simulink model "adsl_sim"  (Simulink 6.0)
settings: Solver=ode45  SolverMode=SingleTasking  StartTime=0.0  StopTime=2  RelTol=1e-3
PreLoadFcn:
  | % variables are initialized through the Model Workspace
model workspace: external: M-Code (data not in the file)
values from neighbouring files (symbols this model uses):
  H = conv2(chCoeff',W)    [eq_computecostfcn.m]
undefined symbols (not defined in the file or in its folder): b, rsgenpoly, slcm
libraries: commdigbbndam2 x512, simulink x37, commutil2 x8, commblkcod2 x4, commsequence2 x4, commsink2 x4, commcrc2 x4, commcnvintrlv2 x2, dspxfrm3 x2, dspsrcs4 x2, dspsigattribs x1, dspmtrx3 x1
(part 1 of 5)
Description:
  | 256 Channel Discrete Multi-Tone Signaling as used in ADSL
CloseFcn:
  | clear adslSigsOut
  | clear global GF_TABLE1 GF_TABLE2 GF_TABLE_M GF_TABLE_PRIM_POLY
settings Model: CovMetricSettings=d  Creator=mikem  LastModifiedBy=akansal  ExtModeAutoUpdateStatusClock=off  BufferReuse=off  ProdHWDeviceType=Specified
settings DataIOCC: SaveOutput=off  SaveTime=off  SignalLoggingName=adslSigsOut
settings OptimizationCC: BlockReduction=off  BooleanDataType=off  OptimizeBlockIOStorage=off  BufferReuse=off  LocalBlockOutputs=off
settings DebuggingCC: CheckExecutionContextPreStartOutputMsg=on  CheckExecutionContextRuntimeOutputMsg=on  SolverPrmCheckMsg=none
settings HardwareCC: ProdHWDeviceType=Specified
settings ModelReferenceCC: UpdateModelReferenceTargets=IfOutOfDate
settings GRTTargetCC: LifeSpan=inf
settings SFSimCC: SFSimApplyToAllLibs=on  SFSimBuildMode=Incremental

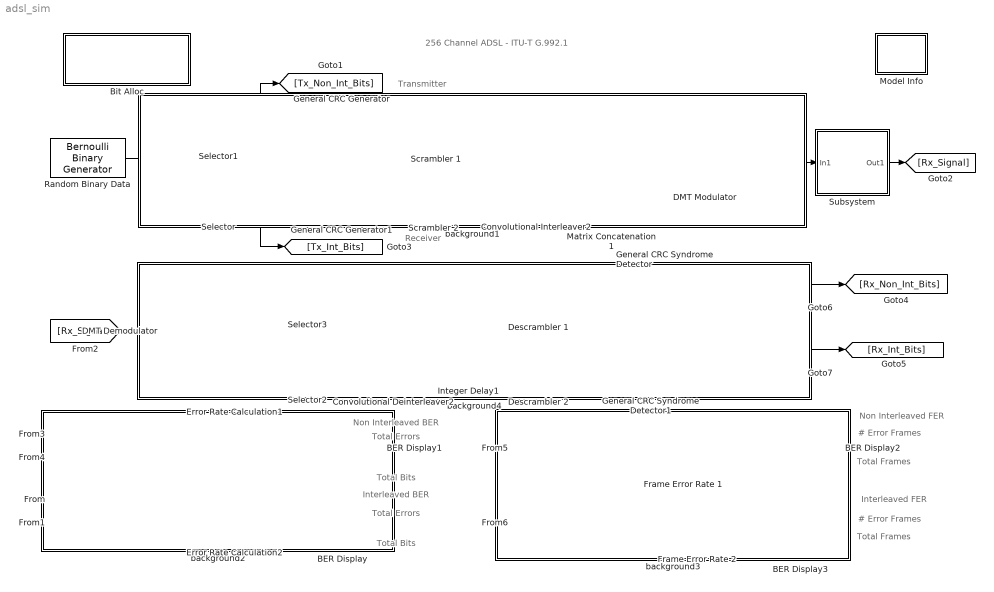
== system adsl_sim ==
  note: Transmitter
  note: Receiver
  note: 256 Channel ADSL - ITU-T G.992.1
  note: Total Bits
  note: Total Errors
  note: Non Interleaved BER
  note: Total Bits
  note: Total Errors
  note: Interleaved BER
  note: # Error Frames
  note: Total Frames
  note: Interleaved FER
  note: # Error Frames
  note: Total Frames
  note: Non Interleaved FER
  BER Display{,1..3} (4 alike) : Display
  Bit Alloc : Subsystem  EnableExecutionContextPropagation=on
      settings: OpenFcn=load('bit_allocation'),plot(b),axis([0 257 1 11]),title('Bit Allocations'),xlabel('Channel'),ylabel('No. Bits')
      mask Display: disp('Load and Plot\nBit Allocation Vector')
  Convolutional Deinterleaver2 : commcnvintrlv2/Convolutional Deinterleaver  N=5  B=2  ic=0
  Convolutional Interleaver2 : commcnvintrlv2/Convolutional Interleaver  N=5  B=2  ic=0
  DMT Demodulator : Subsystem  EnableExecutionContextPropagation=on
      mask Display: disp('DMT\nDemodulator')
  DMT Modulator : Subsystem  EnableExecutionContextPropagation=on
      mask Display: disp('DMT\nModulator')
  Descrambler 1 : Subsystem  EnableExecutionContextPropagation=on
      mask Display: disp('Descrambler\n & FEC');
  Descrambler 2 : Subsystem  EnableExecutionContextPropagation=on
      mask Display: disp('Descrambler\n & FEC');
  Error Rate Calculation1 : commsink2/Error Rate Calculation  N=0  st_delay=0  cp_mode=Entire frame  subframe=[]  PMode=Port  WsName=ErrorVec  RsMode2=off  stop=off  numErr=100  maxBits=1000
  Error Rate Calculation2 : commsink2/Error Rate Calculation  N=776  st_delay=0  cp_mode=Entire frame  subframe=[]  PMode=Port  WsName=ErrorVec  RsMode2=off  stop=off  numErr=100  maxBits=1000
  Frame Error Rate 1 : Subsystem  EnableExecutionContextPropagation=on
      mask Display: disp('Frame Error Rate\n Calculation');
  Frame Error Rate 2 : Subsystem  EnableExecutionContextPropagation=on
      mask Display: disp('Frame Error Rate\n Calculation');
  General CRC Generator : commcrc2/General CRC Generator  genPoly=[1 0 0 0 1 1 1 0 1]  iniStates=[0]  numChecksums=1
  General CRC Generator1 : commcrc2/General CRC Generator  genPoly=[1 0 0 0 1 1 1 0 1]  iniStates=[0]  numChecksums=1
  General CRC Syndrome Detector : commcrc2/General CRC Syndrome Detector  genPoly=[1 0 0 0 1 1 1 0 1]  iniStates=[0]  numChecksums=1
  General CRC Syndrome Detector1 : commcrc2/General CRC Syndrome Detector  genPoly=[1 0 0 0 1 1 1 0 1]  iniStates=[0]  numChecksums=1
  Integer Delay1 : dspsigops/Delay  dly_unit=Samples  delay=800  ic_detail=off  dif_ic_for_ch=off  dif_ic_for_dly=off  ic=0  reset_popup=None
  Matrix Concatenation1 : simulink/Math Operations/Matrix Concatenation  numInports=2  catMethod=Vertical
  Model Info : Subsystem  LoadFcn=slcm LoadBlock;  InitFcn=slcm('UpdateAllCMBlocksInThisModelInit')  EnableExecutionContextPropagation=on  mask(CMBlock){InitialSaveTempField=, InitialBlockCM=none, BlockCM=none, Frame=on, SaveTempField=, DisplayStringWithTags=Info, MaskDisplayString=Info, HorizontalTextAlignment=Center, LeftAlignmentValue=0.5, SourceBlockDiagram=adsl_sim, TagMaxNumber=20, CMTag1=, CMTag2=, CMTag3=, CMTag4=, CMTag5=, CMTag6=, CMTag7=, CMTag8=, CMTag9=, CMTag10=, CMTag11=, CMTag12=, CMTag13=, CMTag14=, CMTag15=, CMTag16=, CMTag17=, CMTag18=, CMTag19=, CMTag20=}
      mask help: This block allows revision control information to be displayed within the model.
      settings: CopyFcn=slcm CopyBlock;  DeleteFcn=slcm Cancel;  PostSaveFcn=slcm('UpdateAllCMBlocksInThisModel')  NameChangeFcn=slcm Rename;  OpenFcn=commdemohelp;
      mask Display: text(str2num(LeftAlignmentValue), 0.5, MaskDisplayString, 'HorizontalAlignment', HorizontalTextAlignment)
  Random Binary Data : commrandsrc2/Bernoulli Binary Generator  P=0.5  seed=4321  Ts=(1/4000)/1552  frameBased=on  sampPerFrame=1552  orient=off
  Scrambler 1 : Subsystem  EnableExecutionContextPropagation=on
      mask Display: disp('Scrambler\n & FEC');
  Scrambler 2 : Subsystem  EnableExecutionContextPropagation=on
      mask Display: disp('Scrambler \n & FEC');
  Selector : Selector  Elements=[777:1552]  InputPortWidth=1552
  Selector1 : Selector  Elements=[1:776]  InputPortWidth=1552
  Selector2 : Selector  Elements=[841:1680]  InputPortWidth=1680
  Selector3 : Selector  Elements=[1:840]  InputPortWidth=1680
  Subsystem : Subsystem  EnableExecutionContextPropagation=on
      mask Type: telchannel
      mask Display: disp('Telephone\nLine');
  background1 : Subsystem  EnableExecutionContextPropagation=on
      mask Display: disp('')
  background2 : Subsystem  EnableExecutionContextPropagation=on
      mask Display: disp('')
  background3 : Subsystem  EnableExecutionContextPropagation=on
      mask Display: disp('')
  background4 : Subsystem  EnableExecutionContextPropagation=on
      mask Display: disp('')
  wires:
  Error Rate Calculation2/1 -> BER Display/1
  DMT Modulator/1(Out) -> Subsystem/1(In1)
  Scrambler 1/1(Out1) -> Matrix Concatenation1/1
  Matrix Concatenation1/1 -> DMT Modulator/1(In)
  Selector3/1 -> Descrambler 1/1(In1)
  Scrambler 2/1(Out1) -> Convolutional Interleaver2/1
  Convolutional Interleaver2/1 -> Matrix Concatenation1/2
  Selector2/1 -> Convolutional Deinterleaver2/1
  Convolutional Deinterleaver2/1 -> Integer Delay1/1
  General CRC Generator1/1 -> Scrambler 2/1(In1)
  Selector/1 -> [Tx_Int_Bits], General CRC Generator1/1
  Selector1/1 -> [Tx_Non_Int_Bits], General CRC Generator/1
  General CRC Generator/1 -> Scrambler 1/1(In1)
  General CRC Syndrome Detector/1 -> [Rx_Non_Int_Bits]
  General CRC Syndrome Detector1/1 -> [Rx_Int_Bits]
  Descrambler 2/1(Out1) -> General CRC Syndrome Detector1/1
  Descrambler 1/1(Out1) -> General CRC Syndrome Detector/1
  General CRC Syndrome Detector1/2 -> [CRC_syndrome2]
  General CRC Syndrome Detector/2 -> [CRC_syndrome1]
  [Tx_Int_Bits] -> Error Rate Calculation2/1
  [Rx_Int_Bits] -> Error Rate Calculation2/2
  Subsystem/1(Out1) -> [Rx_Signal]
  [Rx_Signal] -> DMT Demodulator/1(In)
  Random Binary Data/1 -> Selector/1, Selector1/1
  Error Rate Calculation1/1 -> BER Display1/1
  [Tx_Non_Int_Bits] -> Error Rate Calculation1/1
  [Rx_Non_Int_Bits] -> Error Rate Calculation1/2
  DMT Demodulator/1(Out) -> Selector3/1, Selector2/1
  Frame Error Rate 1/1(Out1) -> BER Display2/1
  [CRC_syndrome1] -> Frame Error Rate 1/1(In1)
  Frame Error Rate 2/1(Out1) -> BER Display3/1
  [CRC_syndrome2] -> Frame Error Rate 2/1(In1)
  Integer Delay1/1 -> Descrambler 2/1(In1)

== system adsl_sim/Bit Alloc ==

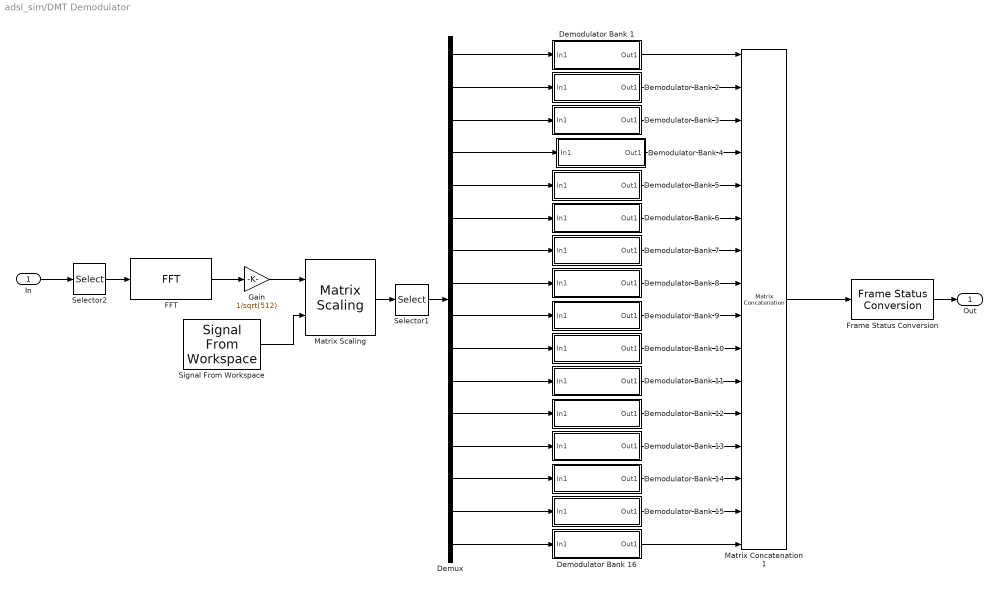
== system adsl_sim/DMT Demodulator ==
  In : Inport  LatchInput=off
  Demodulator Bank 1 : Subsystem  EnableExecutionContextPropagation=on  mask(Demodulator Bank){offset=16*0}
      mask prompts: offset "Index offset:"
      mask help: Bank of sixteen demodulators for use in DMT. Each demodulator in the bank is a Rectangular QAM demodulator. The M-ary number for each demodulator is taken from a workspace variable b. The Index offset parameter determines which sixteen consecutive values from b to use for this bank of demodulators.
      mask Display: disp('Demodulator\nBank');
  Demodulator Bank 10 : Subsystem  EnableExecutionContextPropagation=on  mask(Demodulator Bank){offset=16*9}
      mask prompts: offset "Index offset:"
      mask help: Bank of sixteen demodulators for use in DMT. Each demodulator in the bank is a Rectangular QAM demodulator. The M-ary number for each demodulator is taken from a workspace variable b. The Index offset parameter determines which sixteen consecutive values from b to use for this bank of demodulators.
      mask Display: disp('Demodulator\nBank');
  Demodulator Bank 11 : Subsystem  EnableExecutionContextPropagation=on  mask(Demodulator Bank){offset=16*10}
      mask prompts: offset "Index offset:"
      mask help: Bank of sixteen demodulators for use in DMT. Each demodulator in the bank is a Rectangular QAM demodulator. The M-ary number for each demodulator is taken from a workspace variable b. The Index offset parameter determines which sixteen consecutive values from b to use for this bank of demodulators.
      mask Display: disp('Demodulator\nBank');
  Demodulator Bank 12 : Subsystem  EnableExecutionContextPropagation=on  mask(Demodulator Bank){offset=16*11}
      mask prompts: offset "Index offset:"
      mask help: Bank of sixteen demodulators for use in DMT. Each demodulator in the bank is a Rectangular QAM demodulator. The M-ary number for each demodulator is taken from a workspace variable b. The Index offset parameter determines which sixteen consecutive values from b to use for this bank of demodulators.
      mask Display: disp('Demodulator\nBank');
  Demodulator Bank 13 : Subsystem  EnableExecutionContextPropagation=on  mask(Demodulator Bank){offset=16*12}
      mask prompts: offset "Index offset:"
      mask help: Bank of sixteen demodulators for use in DMT. Each demodulator in the bank is a Rectangular QAM demodulator. The M-ary number for each demodulator is taken from a workspace variable b. The Index offset parameter determines which sixteen consecutive values from b to use for this bank of demodulators.
      mask Display: disp('Demodulator\nBank');
  Demodulator Bank 14 : Subsystem  EnableExecutionContextPropagation=on  mask(Demodulator Bank){offset=16*13}
      mask prompts: offset "Index offset:"
      mask help: Bank of sixteen demodulators for use in DMT. Each demodulator in the bank is a Rectangular QAM demodulator. The M-ary number for each demodulator is taken from a workspace variable b. The Index offset parameter determines which sixteen consecutive values from b to use for this bank of demodulators.
      mask Display: disp('Demodulator\nBank');
  Demodulator Bank 15 : Subsystem  EnableExecutionContextPropagation=on  mask(Demodulator Bank){offset=16*14}
      mask prompts: offset "Index offset:"
      mask help: Bank of sixteen demodulators for use in DMT. Each demodulator in the bank is a Rectangular QAM demodulator. The M-ary number for each demodulator is taken from a workspace variable b. The Index offset parameter determines which sixteen consecutive values from b to use for this bank of demodulators.
      mask Display: disp('Demodulator\nBank');
  Demodulator Bank 16 : Subsystem  EnableExecutionContextPropagation=on  mask(Demodulator Bank){offset=16*15}
      mask prompts: offset "Index offset:"
      mask help: Bank of sixteen demodulators for use in DMT. Each demodulator in the bank is a Rectangular QAM demodulator. The M-ary number for each demodulator is taken from a workspace variable b. The Index offset parameter determines which sixteen consecutive values from b to use for this bank of demodulators.
      mask Display: disp('Demodulator\nBank');
  Demodulator Bank 2 : Subsystem  EnableExecutionContextPropagation=on  mask(Demodulator Bank){offset=16*1}
      mask prompts: offset "Index offset:"
      mask help: Bank of sixteen demodulators for use in DMT. Each demodulator in the bank is a Rectangular QAM demodulator. The M-ary number for each demodulator is taken from a workspace variable b. The Index offset parameter determines which sixteen consecutive values from b to use for this bank of demodulators.
      mask Display: disp('Demodulator\nBank');
  Demodulator Bank 3 : Subsystem  EnableExecutionContextPropagation=on  mask(Demodulator Bank){offset=16*2}
      mask prompts: offset "Index offset:"
      mask help: Bank of sixteen demodulators for use in DMT. Each demodulator in the bank is a Rectangular QAM demodulator. The M-ary number for each demodulator is taken from a workspace variable b. The Index offset parameter determines which sixteen consecutive values from b to use for this bank of demodulators.
      mask Display: disp('Demodulator\nBank');
  Demodulator Bank 4 : Subsystem  EnableExecutionContextPropagation=on  mask(Demodulator Bank){offset=16*3}
      mask prompts: offset "Index offset:"
      mask help: Bank of sixteen demodulators for use in DMT. Each demodulator in the bank is a Rectangular QAM demodulator. The M-ary number for each demodulator is taken from a workspace variable b. The Index offset parameter determines which sixteen consecutive values from b to use for this bank of demodulators.
      mask Display: disp('Demodulator\nBank');
  Demodulator Bank 5 : Subsystem  EnableExecutionContextPropagation=on  mask(Demodulator Bank){offset=16*4}
      mask prompts: offset "Index offset:"
      mask help: Bank of sixteen demodulators for use in DMT. Each demodulator in the bank is a Rectangular QAM demodulator. The M-ary number for each demodulator is taken from a workspace variable b. The Index offset parameter determines which sixteen consecutive values from b to use for this bank of demodulators.
      mask Display: disp('Demodulator\nBank');
  Demodulator Bank 6 : Subsystem  EnableExecutionContextPropagation=on  mask(Demodulator Bank){offset=16*5}
      mask prompts: offset "Index offset:"
      mask help: Bank of sixteen demodulators for use in DMT. Each demodulator in the bank is a Rectangular QAM demodulator. The M-ary number for each demodulator is taken from a workspace variable b. The Index offset parameter determines which sixteen consecutive values from b to use for this bank of demodulators.
      mask Display: disp('Demodulator\nBank');
  Demodulator Bank 7 : Subsystem  EnableExecutionContextPropagation=on  mask(Demodulator Bank){offset=16*6}
      mask prompts: offset "Index offset:"
      mask help: Bank of sixteen demodulators for use in DMT. Each demodulator in the bank is a Rectangular QAM demodulator. The M-ary number for each demodulator is taken from a workspace variable b. The Index offset parameter determines which sixteen consecutive values from b to use for this bank of demodulators.
      mask Display: disp('Demodulator\nBank');
  Demodulator Bank 8 : Subsystem  EnableExecutionContextPropagation=on  mask(Demodulator Bank){offset=16*7}
      mask prompts: offset "Index offset:"
      mask help: Bank of sixteen demodulators for use in DMT. Each demodulator in the bank is a Rectangular QAM demodulator. The M-ary number for each demodulator is taken from a workspace variable b. The Index offset parameter determines which sixteen consecutive values from b to use for this bank of demodulators.
      mask Display: disp('Demodulator\nBank');
  Demodulator Bank 9 : Subsystem  EnableExecutionContextPropagation=on  mask(Demodulator Bank){offset=16*8}
      mask prompts: offset "Index offset:"
      mask help: Bank of sixteen demodulators for use in DMT. Each demodulator in the bank is a Rectangular QAM demodulator. The M-ary number for each demodulator is taken from a workspace variable b. The Index offset parameter determines which sixteen consecutive values from b to use for this bank of demodulators.
      mask Display: disp('Demodulator\nBank');
  Demux : Demux  Outputs=16
  FFT : dspxfrm3/FFT  CompMethod=Table lookup  TableOpt=Speed  BitRevOrder=off  SkipNorm=off  firstCoeffMode=Binary point scaling  firstCoeffWordLength=16  firstCoeffFracLength=15  roundingMode=Floor  overflowMode=off
  Frame Status Conversion : dspsigattribs/Frame Status Conversion  growRefPort=off  outframe=Frame-based
  Gain : Gain  Gain=1/sqrt(512)  SaturateOnIntegerOverflow=on
  Matrix Concatenation1 : simulink/Math Operations/Matrix Concatenation  numInports=16  catMethod=Vertical
  Matrix Scaling : dspmtrx3/Matrix Scaling  mode=Scale rows (D*A)  D_Source=Input port  D_VectFromMask=[0.5 0.25]  roundingMode=Floor  overflowMode=off
  Selector1 : Selector  Elements=[1:256]  InputPortWidth=2*length(b)
  Selector2 : Selector  Elements=[102:613]  InputPortWidth=2*length(b)+101
  Signal From Workspace : dspsrcs4/Signal From Workspace  X=1./H  Ts=1/4000/512  nsamps=512  OutputAfterFinalValue=Cyclic repetition
  Out : Outport
  wires:
  Frame Status Conversion/1 -> Out/1
  Demodulator Bank 16/1(Out1) -> Matrix Concatenation1/16
  Demodulator Bank 15/1(Out1) -> Matrix Concatenation1/15
  Demodulator Bank 14/1(Out1) -> Matrix Concatenation1/14
  Demodulator Bank 13/1(Out1) -> Matrix Concatenation1/13
  Demodulator Bank 12/1(Out1) -> Matrix Concatenation1/12
  Demodulator Bank 11/1(Out1) -> Matrix Concatenation1/11
  Demodulator Bank 10/1(Out1) -> Matrix Concatenation1/10
  Demodulator Bank 9/1(Out1) -> Matrix Concatenation1/9
  Demodulator Bank 8/1(Out1) -> Matrix Concatenation1/8
  Demodulator Bank 7/1(Out1) -> Matrix Concatenation1/7
  Demodulator Bank 6/1(Out1) -> Matrix Concatenation1/6
  Demodulator Bank 5/1(Out1) -> Matrix Concatenation1/5
  Demodulator Bank 4/1(Out1) -> Matrix Concatenation1/4
  Demodulator Bank 3/1(Out1) -> Matrix Concatenation1/3
  Demux/16 -> Demodulator Bank 16/1(In1)
  Demux/15 -> Demodulator Bank 15/1(In1)
  Demux/14 -> Demodulator Bank 14/1(In1)
  Demux/13 -> Demodulator Bank 13/1(In1)
  Demux/12 -> Demodulator Bank 12/1(In1)
  Demux/11 -> Demodulator Bank 11/1(In1)
  Demux/10 -> Demodulator Bank 10/1(In1)
  Demux/9 -> Demodulator Bank 9/1(In1)
  Demux/8 -> Demodulator Bank 8/1(In1)
  Demux/7 -> Demodulator Bank 7/1(In1)
  Demux/6 -> Demodulator Bank 6/1(In1)
  Demux/5 -> Demodulator Bank 5/1(In1)
  Demux/4 -> Demodulator Bank 4/1(In1)
  Demux/3 -> Demodulator Bank 3/1(In1)
  Demux/1 -> Demodulator Bank 1/1(In1)
  Demodulator Bank 1/1(Out1) -> Matrix Concatenation1/1
  Matrix Concatenation1/1 -> Frame Status Conversion/1
  Signal From Workspace/1 -> Matrix Scaling/2
  Matrix Scaling/1 -> Selector1/1
  Selector1/1 -> Demux/1
  Selector2/1 -> FFT/1
  In/1 -> Selector2/1
  Gain/1 -> Matrix Scaling/1
  FFT/1 -> Gain/1
  Demux/2 -> Demodulator Bank 2/1(In1)
  Demodulator Bank 2/1(Out1) -> Matrix Concatenation1/2

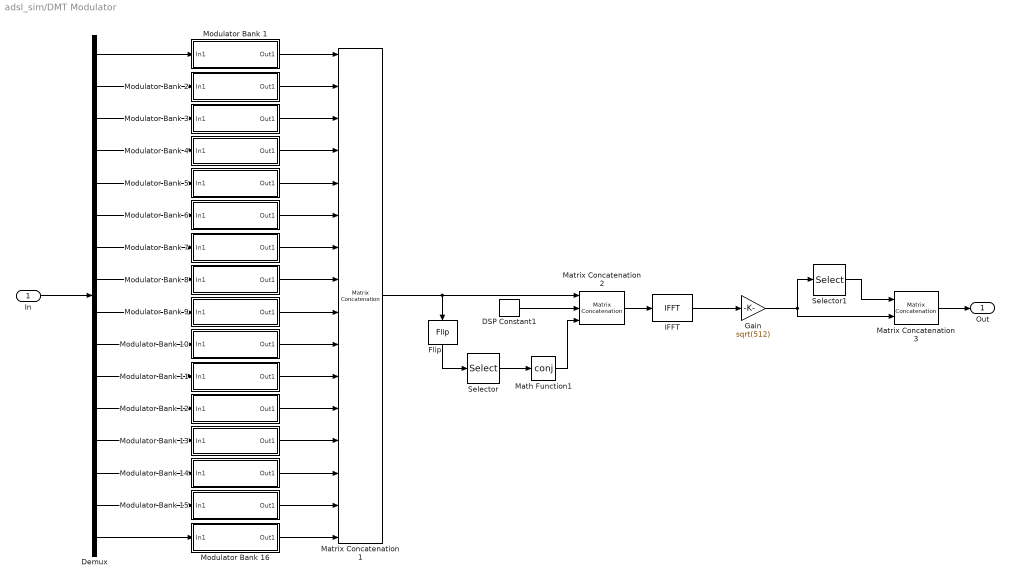
== system adsl_sim/DMT Modulator ==
  In : Inport  LatchInput=off
  DSP Constant1 : dspsrcs4/DSP Constant  Value=0  SampleMode=Discrete  discreteOutput=Frame-based  continuousOutput=Sample-based  sampTime=(1/4000)  framePeriod=(1/4000)  dataType=Inherit from 'Constant value'  wordLen=16  udDataType=sfix(16)  fracBitsMode=Best precision  numFracBits=15  InterpretAs1D=off  Ts=(1/4000)  FramebasedOutput=on
  Demux : Demux  Outputs=sum(reshape(b,16,16))
  Flip : dspindex/Flip  Orientation=down  dim=Columns
  Gain : Gain  Gain=sqrt(512)  SaturateOnIntegerOverflow=on
  IFFT : dspxfrm3/IFFT  CompMethod=Table lookup  TableOpt=Speed  BitRevOrder=off  cs_in=on  SkipNorm=off  mode=Real  firstCoeffMode=Binary point scaling  firstCoeffWordLength=16  firstCoeffFracLength=15  roundingMode=Floor  overflowMode=off
  Math Function1 : Math  Operator=conj  SaturateOnIntegerOverflow=on
  Matrix Concatenation1 : simulink/Math Operations/Matrix Concatenation  numInports=16  catMethod=Vertical
  Matrix Concatenation2 : simulink/Math Operations/Matrix Concatenation  numInports=3  catMethod=Vertical
  Matrix Concatenation3 : simulink/Math Operations/Matrix Concatenation  numInports=2  catMethod=Vertical
  Modulator Bank 1 : Subsystem  EnableExecutionContextPropagation=on  mask(Modulator Bank){offset=16*0}
      mask prompts: offset "Index offset:"
      mask help: Bank of sixteen modulators for use in DMT. Each modulator in the bank is a Rectangular QAM modulator. The M-ary number for each modulator is taken from a workspace variable b. The Index offset parameter determines which sixteen consecutive values from b to use for this bank of modulators.
      mask Display: disp('Modulator\nBank');
  Modulator Bank 10 : Subsystem  EnableExecutionContextPropagation=on  mask(Modulator Bank){offset=16*9}
      mask prompts: offset "Index offset:"
      mask help: Bank of sixteen modulators for use in DMT. Each modulator in the bank is a Rectangular QAM modulator. The M-ary number for each modulator is taken from a workspace variable b. The Index offset parameter determines which sixteen consecutive values from b to use for this bank of modulators.
      mask Display: disp('Modulator\nBank');
  Modulator Bank 11 : Subsystem  EnableExecutionContextPropagation=on  mask(Modulator Bank){offset=16*10}
      mask prompts: offset "Index offset:"
      mask help: Bank of sixteen modulators for use in DMT. Each modulator in the bank is a Rectangular QAM modulator. The M-ary number for each modulator is taken from a workspace variable b. The Index offset parameter determines which sixteen consecutive values from b to use for this bank of modulators.
      mask Display: disp('Modulator\nBank');
  Modulator Bank 12 : Subsystem  EnableExecutionContextPropagation=on  mask(Modulator Bank){offset=16*11}
      mask prompts: offset "Index offset:"
      mask help: Bank of sixteen modulators for use in DMT. Each modulator in the bank is a Rectangular QAM modulator. The M-ary number for each modulator is taken from a workspace variable b. The Index offset parameter determines which sixteen consecutive values from b to use for this bank of modulators.
      mask Display: disp('Modulator\nBank');
  Modulator Bank 13 : Subsystem  EnableExecutionContextPropagation=on  mask(Modulator Bank){offset=16*12}
      mask prompts: offset "Index offset:"
      mask help: Bank of sixteen modulators for use in DMT. Each modulator in the bank is a Rectangular QAM modulator. The M-ary number for each modulator is taken from a workspace variable b. The Index offset parameter determines which sixteen consecutive values from b to use for this bank of modulators.
      mask Display: disp('Modulator\nBank');
  Modulator Bank 14 : Subsystem  EnableExecutionContextPropagation=on  mask(Modulator Bank){offset=16*13}
      mask prompts: offset "Index offset:"
      mask help: Bank of sixteen modulators for use in DMT. Each modulator in the bank is a Rectangular QAM modulator. The M-ary number for each modulator is taken from a workspace variable b. The Index offset parameter determines which sixteen consecutive values from b to use for this bank of modulators.
      mask Display: disp('Modulator\nBank');
  Modulator Bank 15 : Subsystem  EnableExecutionContextPropagation=on  mask(Modulator Bank){offset=16*14}
      mask prompts: offset "Index offset:"
      mask help: Bank of sixteen modulators for use in DMT. Each modulator in the bank is a Rectangular QAM modulator. The M-ary number for each modulator is taken from a workspace variable b. The Index offset parameter determines which sixteen consecutive values from b to use for this bank of modulators.
      mask Display: disp('Modulator\nBank');
  Modulator Bank 16 : Subsystem  EnableExecutionContextPropagation=on  mask(Modulator Bank){offset=16*15}
      mask prompts: offset "Index offset:"
      mask help: Bank of sixteen modulators for use in DMT. Each modulator in the bank is a Rectangular QAM modulator. The M-ary number for each modulator is taken from a workspace variable b. The Index offset parameter determines which sixteen consecutive values from b to use for this bank of modulators.
      mask Display: disp('Modulator\nBank');
  Modulator Bank 2 : Subsystem  EnableExecutionContextPropagation=on  mask(Modulator Bank){offset=16*1}
      mask prompts: offset "Index offset:"
      mask help: Bank of sixteen modulators for use in DMT. Each modulator in the bank is a Rectangular QAM modulator. The M-ary number for each modulator is taken from a workspace variable b. The Index offset parameter determines which sixteen consecutive values from b to use for this bank of modulators.
      mask Display: disp('Modulator\nBank');
  Modulator Bank 3 : Subsystem  EnableExecutionContextPropagation=on  mask(Modulator Bank){offset=16*2}
      mask prompts: offset "Index offset:"
      mask help: Bank of sixteen modulators for use in DMT. Each modulator in the bank is a Rectangular QAM modulator. The M-ary number for each modulator is taken from a workspace variable b. The Index offset parameter determines which sixteen consecutive values from b to use for this bank of modulators.
      mask Display: disp('Modulator\nBank');
  Modulator Bank 4 : Subsystem  EnableExecutionContextPropagation=on  mask(Modulator Bank){offset=16*3}
      mask prompts: offset "Index offset:"
      mask help: Bank of sixteen modulators for use in DMT. Each modulator in the bank is a Rectangular QAM modulator. The M-ary number for each modulator is taken from a workspace variable b. The Index offset parameter determines which sixteen consecutive values from b to use for this bank of modulators.
      mask Display: disp('Modulator\nBank');
  Modulator Bank 5 : Subsystem  EnableExecutionContextPropagation=on  mask(Modulator Bank){offset=16*4}
      mask prompts: offset "Index offset:"
      mask help: Bank of sixteen modulators for use in DMT. Each modulator in the bank is a Rectangular QAM modulator. The M-ary number for each modulator is taken from a workspace variable b. The Index offset parameter determines which sixteen consecutive values from b to use for this bank of modulators.
      mask Display: disp('Modulator\nBank');
  Modulator Bank 6 : Subsystem  EnableExecutionContextPropagation=on  mask(Modulator Bank){offset=16*5}
      mask prompts: offset "Index offset:"
      mask help: Bank of sixteen modulators for use in DMT. Each modulator in the bank is a Rectangular QAM modulator. The M-ary number for each modulator is taken from a workspace variable b. The Index offset parameter determines which sixteen consecutive values from b to use for this bank of modulators.
      mask Display: disp('Modulator\nBank');
  Modulator Bank 7 : Subsystem  EnableExecutionContextPropagation=on  mask(Modulator Bank){offset=16*6}
      mask prompts: offset "Index offset:"
      mask help: Bank of sixteen modulators for use in DMT. Each modulator in the bank is a Rectangular QAM modulator. The M-ary number for each modulator is taken from a workspace variable b. The Index offset parameter determines which sixteen consecutive values from b to use for this bank of modulators.
      mask Display: disp('Modulator\nBank');
  Modulator Bank 8 : Subsystem  EnableExecutionContextPropagation=on  mask(Modulator Bank){offset=16*7}
      mask prompts: offset "Index offset:"
      mask help: Bank of sixteen modulators for use in DMT. Each modulator in the bank is a Rectangular QAM modulator. The M-ary number for each modulator is taken from a workspace variable b. The Index offset parameter determines which sixteen consecutive values from b to use for this bank of modulators.
      mask Display: disp('Modulator\nBank');
  Modulator Bank 9 : Subsystem  EnableExecutionContextPropagation=on  mask(Modulator Bank){offset=16*8}
      mask prompts: offset "Index offset:"
      mask help: Bank of sixteen modulators for use in DMT. Each modulator in the bank is a Rectangular QAM modulator. The M-ary number for each modulator is taken from a workspace variable b. The Index offset parameter determines which sixteen consecutive values from b to use for this bank of modulators.
      mask Display: disp('Modulator\nBank');
  Selector : Selector  Elements=[1:length(b)-1]  InputPortWidth=length(b)
  Selector1 : Selector  Elements=[412:512]  InputPortWidth=2*length(b)
  Out : Outport
  wires:
  Modulator Bank 1/1(Out1) -> Matrix Concatenation1/1
  Demux/1 -> Modulator Bank 1/1(In1)
  Demux/2 -> Modulator Bank 2/1(In1)
  In/1 -> Demux/1
  Demux/3 -> Modulator Bank 3/1(In1)
  Demux/4 -> Modulator Bank 4/1(In1)
  Demux/5 -> Modulator Bank 5/1(In1)
  Demux/6 -> Modulator Bank 6/1(In1)
  Demux/7 -> Modulator Bank 7/1(In1)
  Demux/8 -> Modulator Bank 8/1(In1)
  Demux/9 -> Modulator Bank 9/1(In1)
  Demux/10 -> Modulator Bank 10/1(In1)
  Demux/11 -> Modulator Bank 11/1(In1)
  Demux/12 -> Modulator Bank 12/1(In1)
  Demux/13 -> Modulator Bank 13/1(In1)
  Demux/14 -> Modulator Bank 14/1(In1)
  Demux/15 -> Modulator Bank 15/1(In1)
  Demux/16 -> Modulator Bank 16/1(In1)
  Modulator Bank 2/1(Out1) -> Matrix Concatenation1/2
  Modulator Bank 3/1(Out1) -> Matrix Concatenation1/3
  Modulator Bank 4/1(Out1) -> Matrix Concatenation1/4
  Modulator Bank 5/1(Out1) -> Matrix Concatenation1/5
  Modulator Bank 6/1(Out1) -> Matrix Concatenation1/6
  Modulator Bank 7/1(Out1) -> Matrix Concatenation1/7
  Modulator Bank 8/1(Out1) -> Matrix Concatenation1/8
  Modulator Bank 9/1(Out1) -> Matrix Concatenation1/9
  Modulator Bank 10/1(Out1) -> Matrix Concatenation1/10
  Modulator Bank 11/1(Out1) -> Matrix Concatenation1/11
  Modulator Bank 12/1(Out1) -> Matrix Concatenation1/12
  Modulator Bank 13/1(Out1) -> Matrix Concatenation1/13
  Modulator Bank 14/1(Out1) -> Matrix Concatenation1/14
  Modulator Bank 15/1(Out1) -> Matrix Concatenation1/15
  Modulator Bank 16/1(Out1) -> Matrix Concatenation1/16
  Matrix Concatenation2/1 -> IFFT/1
  Selector/1 -> Math Function1/1
  Flip/1 -> Selector/1
  Math Function1/1 -> Matrix Concatenation2/3
  DSP Constant1/1 -> Matrix Concatenation2/2
  Matrix Concatenation1/1 -> Flip/1, Matrix Concatenation2/1
  Selector1/1 -> Matrix Concatenation3/1
  Matrix Concatenation3/1 -> Out/1
  IFFT/1 -> Gain/1
  Gain/1 -> Matrix Concatenation3/2, Selector1/1

== system adsl_sim/Descrambler 1 ==
  In1 : Inport  LatchInput=off
  (120,112) Shortened RS Decoder : commblkcod2/Integer-Output RS Decoder  n=120  k=112  specPrimPoly=off  primPoly=[1 0 1 1]  specGenPoly=off  genPoly=rsgenpoly(7,3)  showNumErr=off
  Bit to Integer Converter : commutil2/Bit to Integer Converter  nbits=7
  Descrambler : commsequence2/Descrambler  M=128  poly=[0 -18 -23]  ini_sta=zeros(23,1)
  Integer to Bit Converter : commutil2/Integer to Bit Converter  nbits=7
  Out1 : Outport
  wires:
  Bit to Integer Converter/1 -> (120,112) Shortened RS Decoder/1
  (120,112) Shortened RS Decoder/1 -> Descrambler/1
  Descrambler/1 -> Integer to Bit Converter/1
  Integer to Bit Converter/1 -> Out1/1
  In1/1 -> Bit to Integer Converter/1

== system adsl_sim/Descrambler 2 ==
  In1 : Inport  LatchInput=off
  (120,112) Shortened RS Decoder : commblkcod2/Integer-Output RS Decoder  n=120  k=112  specPrimPoly=off  primPoly=[1 0 1 1]  specGenPoly=off  genPoly=rsgenpoly(7,3)  showNumErr=off
  Bit to Integer Converter : commutil2/Bit to Integer Converter  nbits=7
  Descrambler : commsequence2/Descrambler  M=128  poly=[0 -18 -23]  ini_sta=zeros(23,1)
  Integer to Bit Converter : commutil2/Integer to Bit Converter  nbits=7
  Out1 : Outport
  wires:
  In1/1 -> Bit to Integer Converter/1
  Integer to Bit Converter/1 -> Out1/1
  Descrambler/1 -> Integer to Bit Converter/1
  (120,112) Shortened RS Decoder/1 -> Descrambler/1
  Bit to Integer Converter/1 -> (120,112) Shortened RS Decoder/1

== system adsl_sim/Frame Error Rate 1 ==
  In1 : Inport  LatchInput=off
  Constant : Constant  Value=0
  Error Rate Calculation3 : commsink2/Error Rate Calculation  N=0  st_delay=0  cp_mode=Entire frame  subframe=[]  PMode=Port  WsName=ErrorVec  RsMode2=off  stop=off  numErr=100  maxBits=1000
  Out1 : Outport
  wires:
  Constant/1 -> Error Rate Calculation3/2
  In1/1 -> Error Rate Calculation3/1
  Error Rate Calculation3/1 -> Out1/1

== system adsl_sim/Frame Error Rate 2 ==
  In1 : Inport  LatchInput=off
  Constant : Constant  Value=0
  Error Rate Calculation3 : commsink2/Error Rate Calculation  N=0  st_delay=0  cp_mode=Entire frame  subframe=[]  PMode=Port  WsName=ErrorVec  RsMode2=off  stop=off  numErr=100  maxBits=1000
  Out1 : Outport
  wires:
  Error Rate Calculation3/1 -> Out1/1
  In1/1 -> Error Rate Calculation3/1
  Constant/1 -> Error Rate Calculation3/2

== system adsl_sim/Model Info ==
  EmptySubsystem : Subsystem  EnableExecutionContextPropagation=on

== system adsl_sim/Scrambler 1 ==
  In1 : Inport  LatchInput=off
  (120,112) Shortened RS Encoder : commblkcod2/Integer-Input RS Encoder  n=120  k=112  specPrimPoly=off  primPoly=[1 0 1 1]  specGenPoly=off  genPoly=rsgenpoly(7,3)
  Bit to Integer Converter : commutil2/Bit to Integer Converter  nbits=7
  Integer to Bit Converter : commutil2/Integer to Bit Converter  nbits=7
  Scrambler : commsequence2/Scrambler  M=128  poly=[0 -18 -23]  ini_sta=zeros(23,1)
  Out1 : Outport
  wires:
  (120,112) Shortened RS Encoder/1 -> Integer to Bit Converter/1
  Scrambler/1 -> (120,112) Shortened RS Encoder/1
  In1/1 -> Bit to Integer Converter/1
  Bit to Integer Converter/1 -> Scrambler/1
  Integer to Bit Converter/1 -> Out1/1

== system adsl_sim/Scrambler 2 ==
  In1 : Inport  LatchInput=off
  (120,112) Shortened RS Encoder : commblkcod2/Integer-Input RS Encoder  n=120  k=112  specPrimPoly=off  primPoly=[1 0 1 1]  specGenPoly=off  genPoly=rsgenpoly(7,3)
  Bit to Integer Converter : commutil2/Bit to Integer Converter  nbits=7
  Integer to Bit Converter : commutil2/Integer to Bit Converter  nbits=7
  Scrambler : commsequence2/Scrambler  M=128  poly=[0 -18 -23]  ini_sta=zeros(23,1)
  Out1 : Outport
  wires:
  Integer to Bit Converter/1 -> Out1/1
  Bit to Integer Converter/1 -> Scrambler/1
  In1/1 -> Bit to Integer Converter/1
  Scrambler/1 -> (120,112) Shortened RS Encoder/1
  (120,112) Shortened RS Encoder/1 -> Integer to Bit Converter/1

== system adsl_sim/Subsystem ==
  In1 : Inport  LatchInput=off
  AWGN Channel2 : commchan2/AWGN Channel  seed=12345  noiseMode="Signal to noise ratio  (Es/No)"  EbNodB=10  EsNodB=25  SNRdB=20  bitsPerSym=1  Ps=1  Tsym=1/4000/613  variance=0.000001
  Digital Filter Design : dsparch4/Digital Filter Design
  Out1 : Outport
  wires:
  In1/1 -> Digital Filter Design/1
  AWGN Channel2/1 -> Out1/1
  Digital Filter Design/1 -> AWGN Channel2/1

== system adsl_sim/background1 ==

== system adsl_sim/background2 ==

== system adsl_sim/background3 ==

== system adsl_sim/background4 ==

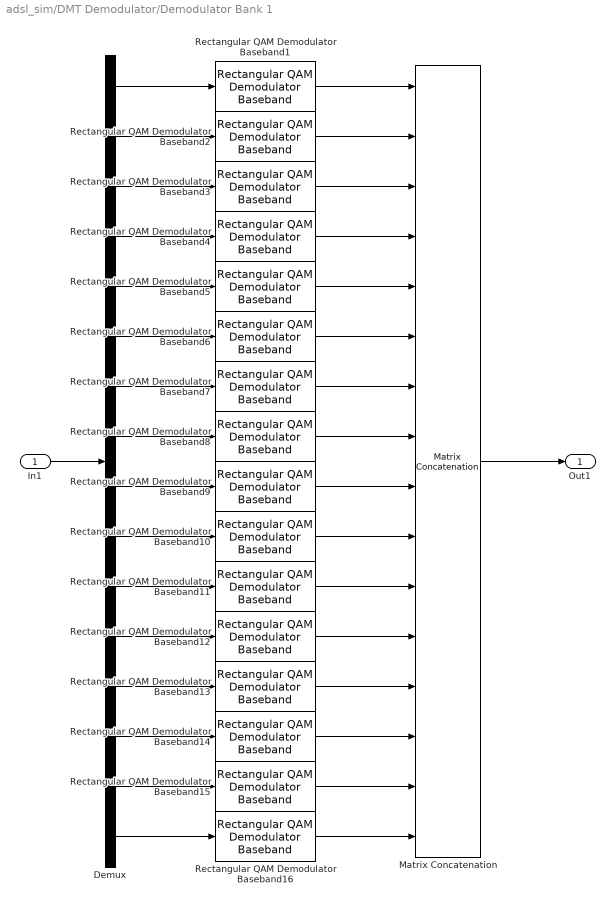
== system adsl_sim/DMT Demodulator/Demodulator Bank 1 ==
  In1 : Inport  LatchInput=off
  Demux : Demux  Outputs=16
  Matrix Concatenation : simulink/Math Operations/Matrix Concatenation  numInports=16  catMethod=Vertical
  Rectangular QAM Demodulator Baseband1 : commdigbbndam2/Rectangular QAM Demodulator Baseband  M=2^b(offset+1)  OutType=Bit  Dec=Gray  PowType=Average Power  MinDist=2  AvgPow=1  PeakPow=1  Ph=0  numSamp=1
  Rectangular QAM Demodulator Baseband10 : commdigbbndam2/Rectangular QAM Demodulator Baseband  M=2^b(offset+10)  OutType=Bit  Dec=Gray  PowType=Average Power  MinDist=2  AvgPow=1  PeakPow=1  Ph=0  numSamp=1
  Rectangular QAM Demodulator Baseband11 : commdigbbndam2/Rectangular QAM Demodulator Baseband  M=2^b(offset+11)  OutType=Bit  Dec=Gray  PowType=Average Power  MinDist=2  AvgPow=1  PeakPow=1  Ph=0  numSamp=1
  Rectangular QAM Demodulator Baseband12 : commdigbbndam2/Rectangular QAM Demodulator Baseband  M=2^b(offset+12)  OutType=Bit  Dec=Gray  PowType=Average Power  MinDist=2  AvgPow=1  PeakPow=1  Ph=0  numSamp=1
  Rectangular QAM Demodulator Baseband13 : commdigbbndam2/Rectangular QAM Demodulator Baseband  M=2^b(offset+13)  OutType=Bit  Dec=Gray  PowType=Average Power  MinDist=2  AvgPow=1  PeakPow=1  Ph=0  numSamp=1
  Rectangular QAM Demodulator Baseband14 : commdigbbndam2/Rectangular QAM Demodulator Baseband  M=2^b(offset+14)  OutType=Bit  Dec=Gray  PowType=Average Power  MinDist=2  AvgPow=1  PeakPow=1  Ph=0  numSamp=1
  Rectangular QAM Demodulator Baseband15 : commdigbbndam2/Rectangular QAM Demodulator Baseband  M=2^b(offset+15)  OutType=Bit  Dec=Gray  PowType=Average Power  MinDist=2  AvgPow=1  PeakPow=1  Ph=0  numSamp=1
  Rectangular QAM Demodulator Baseband16 : commdigbbndam2/Rectangular QAM Demodulator Baseband  M=2^b(offset+16)  OutType=Bit  Dec=Gray  PowType=Average Power  MinDist=2  AvgPow=1  PeakPow=1  Ph=0  numSamp=1
  Rectangular QAM Demodulator Baseband2 : commdigbbndam2/Rectangular QAM Demodulator Baseband  M=2^b(offset+2)  OutType=Bit  Dec=Gray  PowType=Average Power  MinDist=2  AvgPow=1  PeakPow=1  Ph=0  numSamp=1
  Rectangular QAM Demodulator Baseband3 : commdigbbndam2/Rectangular QAM Demodulator Baseband  M=2^b(offset+3)  OutType=Bit  Dec=Gray  PowType=Average Power  MinDist=2  AvgPow=1  PeakPow=1  Ph=0  numSamp=1
  Rectangular QAM Demodulator Baseband4 : commdigbbndam2/Rectangular QAM Demodulator Baseband  M=2^b(offset+4)  OutType=Bit  Dec=Gray  PowType=Average Power  MinDist=2  AvgPow=1  PeakPow=1  Ph=0  numSamp=1
  Rectangular QAM Demodulator Baseband5 : commdigbbndam2/Rectangular QAM Demodulator Baseband  M=2^b(offset+5)  OutType=Bit  Dec=Gray  PowType=Average Power  MinDist=2  AvgPow=1  PeakPow=1  Ph=0  numSamp=1
  Rectangular QAM Demodulator Baseband6 : commdigbbndam2/Rectangular QAM Demodulator Baseband  M=2^b(offset+6)  OutType=Bit  Dec=Gray  PowType=Average Power  MinDist=2  AvgPow=1  PeakPow=1  Ph=0  numSamp=1
  Rectangular QAM Demodulator Baseband7 : commdigbbndam2/Rectangular QAM Demodulator Baseband  M=2^b(offset+7)  OutType=Bit  Dec=Gray  PowType=Average Power  MinDist=2  AvgPow=1  PeakPow=1  Ph=0  numSamp=1
  Rectangular QAM Demodulator Baseband8 : commdigbbndam2/Rectangular QAM Demodulator Baseband  M=2^b(offset+8)  OutType=Bit  Dec=Gray  PowType=Average Power  MinDist=2  AvgPow=1  PeakPow=1  Ph=0  numSamp=1
  Rectangular QAM Demodulator Baseband9 : commdigbbndam2/Rectangular QAM Demodulator Baseband  M=2^b(offset+9)  OutType=Bit  Dec=Gray  PowType=Average Power  MinDist=2  AvgPow=1  PeakPow=1  Ph=0  numSamp=1
  Out1 : Outport
  wires:
  In1/1 -> Demux/1
  Matrix Concatenation/1 -> Out1/1
  Demux/16 -> Rectangular QAM Demodulator Baseband16/1
  Demux/15 -> Rectangular QAM Demodulator Baseband15/1
  Demux/14 -> Rectangular QAM Demodulator Baseband14/1
  Demux/13 -> Rectangular QAM Demodulator Baseband13/1
  Demux/12 -> Rectangular QAM Demodulator Baseband12/1
  Demux/11 -> Rectangular QAM Demodulator Baseband11/1
  Demux/10 -> Rectangular QAM Demodulator Baseband10/1
  Demux/9 -> Rectangular QAM Demodulator Baseband9/1
  Demux/8 -> Rectangular QAM Demodulator Baseband8/1
  Demux/7 -> Rectangular QAM Demodulator Baseband7/1
  Demux/6 -> Rectangular QAM Demodulator Baseband6/1
  Demux/5 -> Rectangular QAM Demodulator Baseband5/1
  Demux/4 -> Rectangular QAM Demodulator Baseband4/1
  Demux/3 -> Rectangular QAM Demodulator Baseband3/1
  Demux/2 -> Rectangular QAM Demodulator Baseband2/1
  Demux/1 -> Rectangular QAM Demodulator Baseband1/1
  Rectangular QAM Demodulator Baseband16/1 -> Matrix Concatenation/16
  Rectangular QAM Demodulator Baseband15/1 -> Matrix Concatenation/15
  Rectangular QAM Demodulator Baseband14/1 -> Matrix Concatenation/14
  Rectangular QAM Demodulator Baseband13/1 -> Matrix Concatenation/13
  Rectangular QAM Demodulator Baseband12/1 -> Matrix Concatenation/12
  Rectangular QAM Demodulator Baseband11/1 -> Matrix Concatenation/11
  Rectangular QAM Demodulator Baseband10/1 -> Matrix Concatenation/10
  Rectangular QAM Demodulator Baseband9/1 -> Matrix Concatenation/9
  Rectangular QAM Demodulator Baseband8/1 -> Matrix Concatenation/8
  Rectangular QAM Demodulator Baseband7/1 -> Matrix Concatenation/7
  Rectangular QAM Demodulator Baseband6/1 -> Matrix Concatenation/6
  Rectangular QAM Demodulator Baseband5/1 -> Matrix Concatenation/5
  Rectangular QAM Demodulator Baseband4/1 -> Matrix Concatenation/4
  Rectangular QAM Demodulator Baseband3/1 -> Matrix Concatenation/3
  Rectangular QAM Demodulator Baseband2/1 -> Matrix Concatenation/2
  Rectangular QAM Demodulator Baseband1/1 -> Matrix Concatenation/1

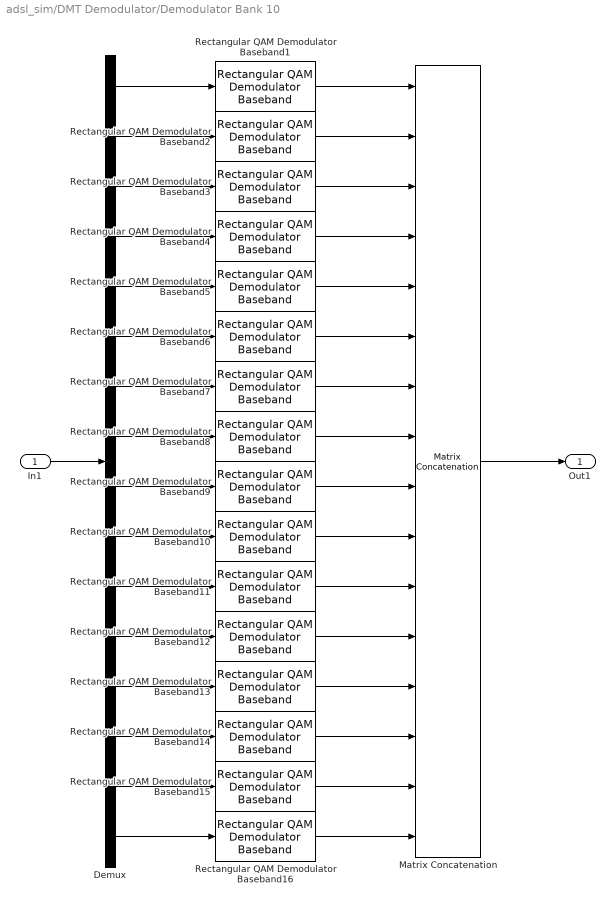
== system adsl_sim/DMT Demodulator/Demodulator Bank 10 ==
  In1 : Inport  LatchInput=off
  Demux : Demux  Outputs=16
  Matrix Concatenation : simulink/Math Operations/Matrix Concatenation  numInports=16  catMethod=Vertical
  Rectangular QAM Demodulator Baseband1 : commdigbbndam2/Rectangular QAM Demodulator Baseband  M=2^b(offset+1)  OutType=Bit  Dec=Gray  PowType=Average Power  MinDist=2  AvgPow=1  PeakPow=1  Ph=0  numSamp=1
  Rectangular QAM Demodulator Baseband10 : commdigbbndam2/Rectangular QAM Demodulator Baseband  M=2^b(offset+10)  OutType=Bit  Dec=Gray  PowType=Average Power  MinDist=2  AvgPow=1  PeakPow=1  Ph=0  numSamp=1
  Rectangular QAM Demodulator Baseband11 : commdigbbndam2/Rectangular QAM Demodulator Baseband  M=2^b(offset+11)  OutType=Bit  Dec=Gray  PowType=Average Power  MinDist=2  AvgPow=1  PeakPow=1  Ph=0  numSamp=1
  Rectangular QAM Demodulator Baseband12 : commdigbbndam2/Rectangular QAM Demodulator Baseband  M=2^b(offset+12)  OutType=Bit  Dec=Gray  PowType=Average Power  MinDist=2  AvgPow=1  PeakPow=1  Ph=0  numSamp=1
  Rectangular QAM Demodulator Baseband13 : commdigbbndam2/Rectangular QAM Demodulator Baseband  M=2^b(offset+13)  OutType=Bit  Dec=Gray  PowType=Average Power  MinDist=2  AvgPow=1  PeakPow=1  Ph=0  numSamp=1
  Rectangular QAM Demodulator Baseband14 : commdigbbndam2/Rectangular QAM Demodulator Baseband  M=2^b(offset+14)  OutType=Bit  Dec=Gray  PowType=Average Power  MinDist=2  AvgPow=1  PeakPow=1  Ph=0  numSamp=1
  Rectangular QAM Demodulator Baseband15 : commdigbbndam2/Rectangular QAM Demodulator Baseband  M=2^b(offset+15)  OutType=Bit  Dec=Gray  PowType=Average Power  MinDist=2  AvgPow=1  PeakPow=1  Ph=0  numSamp=1
  Rectangular QAM Demodulator Baseband16 : commdigbbndam2/Rectangular QAM Demodulator Baseband  M=2^b(offset+16)  OutType=Bit  Dec=Gray  PowType=Average Power  MinDist=2  AvgPow=1  PeakPow=1  Ph=0  numSamp=1
  Rectangular QAM Demodulator Baseband2 : commdigbbndam2/Rectangular QAM Demodulator Baseband  M=2^b(offset+2)  OutType=Bit  Dec=Gray  PowType=Average Power  MinDist=2  AvgPow=1  PeakPow=1  Ph=0  numSamp=1
  Rectangular QAM Demodulator Baseband3 : commdigbbndam2/Rectangular QAM Demodulator Baseband  M=2^b(offset+3)  OutType=Bit  Dec=Gray  PowType=Average Power  MinDist=2  AvgPow=1  PeakPow=1  Ph=0  numSamp=1
  Rectangular QAM Demodulator Baseband4 : commdigbbndam2/Rectangular QAM Demodulator Baseband  M=2^b(offset+4)  OutType=Bit  Dec=Gray  PowType=Average Power  MinDist=2  AvgPow=1  PeakPow=1  Ph=0  numSamp=1
  Rectangular QAM Demodulator Baseband5 : commdigbbndam2/Rectangular QAM Demodulator Baseband  M=2^b(offset+5)  OutType=Bit  Dec=Gray  PowType=Average Power  MinDist=2  AvgPow=1  PeakPow=1  Ph=0  numSamp=1
  Rectangular QAM Demodulator Baseband6 : commdigbbndam2/Rectangular QAM Demodulator Baseband  M=2^b(offset+6)  OutType=Bit  Dec=Gray  PowType=Average Power  MinDist=2  AvgPow=1  PeakPow=1  Ph=0  numSamp=1
  Rectangular QAM Demodulator Baseband7 : commdigbbndam2/Rectangular QAM Demodulator Baseband  M=2^b(offset+7)  OutType=Bit  Dec=Gray  PowType=Average Power  MinDist=2  AvgPow=1  PeakPow=1  Ph=0  numSamp=1
  Rectangular QAM Demodulator Baseband8 : commdigbbndam2/Rectangular QAM Demodulator Baseband  M=2^b(offset+8)  OutType=Bit  Dec=Gray  PowType=Average Power  MinDist=2  AvgPow=1  PeakPow=1  Ph=0  numSamp=1
  Rectangular QAM Demodulator Baseband9 : commdigbbndam2/Rectangular QAM Demodulator Baseband  M=2^b(offset+9)  OutType=Bit  Dec=Gray  PowType=Average Power  MinDist=2  AvgPow=1  PeakPow=1  Ph=0  numSamp=1
  Out1 : Outport
  wires:
  In1/1 -> Demux/1
  Matrix Concatenation/1 -> Out1/1
  Demux/16 -> Rectangular QAM Demodulator Baseband16/1
  Demux/15 -> Rectangular QAM Demodulator Baseband15/1
  Demux/14 -> Rectangular QAM Demodulator Baseband14/1
  Demux/13 -> Rectangular QAM Demodulator Baseband13/1
  Demux/12 -> Rectangular QAM Demodulator Baseband12/1
  Demux/11 -> Rectangular QAM Demodulator Baseband11/1
  Demux/10 -> Rectangular QAM Demodulator Baseband10/1
  Demux/9 -> Rectangular QAM Demodulator Baseband9/1
  Demux/8 -> Rectangular QAM Demodulator Baseband8/1
  Demux/7 -> Rectangular QAM Demodulator Baseband7/1
  Demux/6 -> Rectangular QAM Demodulator Baseband6/1
  Demux/5 -> Rectangular QAM Demodulator Baseband5/1
  Demux/4 -> Rectangular QAM Demodulator Baseband4/1
  Demux/3 -> Rectangular QAM Demodulator Baseband3/1
  Demux/2 -> Rectangular QAM Demodulator Baseband2/1
  Demux/1 -> Rectangular QAM Demodulator Baseband1/1
  Rectangular QAM Demodulator Baseband16/1 -> Matrix Concatenation/16
  Rectangular QAM Demodulator Baseband15/1 -> Matrix Concatenation/15
  Rectangular QAM Demodulator Baseband14/1 -> Matrix Concatenation/14
  Rectangular QAM Demodulator Baseband13/1 -> Matrix Concatenation/13
  Rectangular QAM Demodulator Baseband12/1 -> Matrix Concatenation/12
  Rectangular QAM Demodulator Baseband11/1 -> Matrix Concatenation/11
  Rectangular QAM Demodulator Baseband10/1 -> Matrix Concatenation/10
  Rectangular QAM Demodulator Baseband9/1 -> Matrix Concatenation/9
  Rectangular QAM Demodulator Baseband8/1 -> Matrix Concatenation/8
  Rectangular QAM Demodulator Baseband7/1 -> Matrix Concatenation/7
  Rectangular QAM Demodulator Baseband6/1 -> Matrix Concatenation/6
  Rectangular QAM Demodulator Baseband5/1 -> Matrix Concatenation/5
  Rectangular QAM Demodulator Baseband4/1 -> Matrix Concatenation/4
  Rectangular QAM Demodulator Baseband3/1 -> Matrix Concatenation/3
  Rectangular QAM Demodulator Baseband2/1 -> Matrix Concatenation/2
  Rectangular QAM Demodulator Baseband1/1 -> Matrix Concatenation/1
